simulink model "Laboratory_2_Stateflow"  (R2023b)
settings: Solver=FixedStepAuto  StartTime=0.0  StopTime=1200.0  FixedStep=0.1  RelTol=1e-3
libraries: SignalEditorBlockLib x1
settings Model: PacingRate=10  Creator=cosmi  LastModifiedBy=cosmi

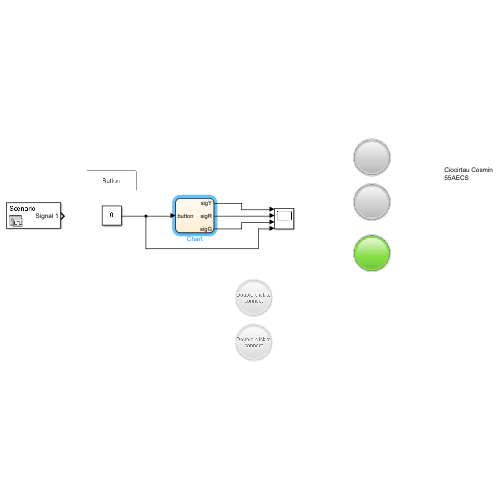
[thumbnail: Simulink's stored preview of the top-level diagram]
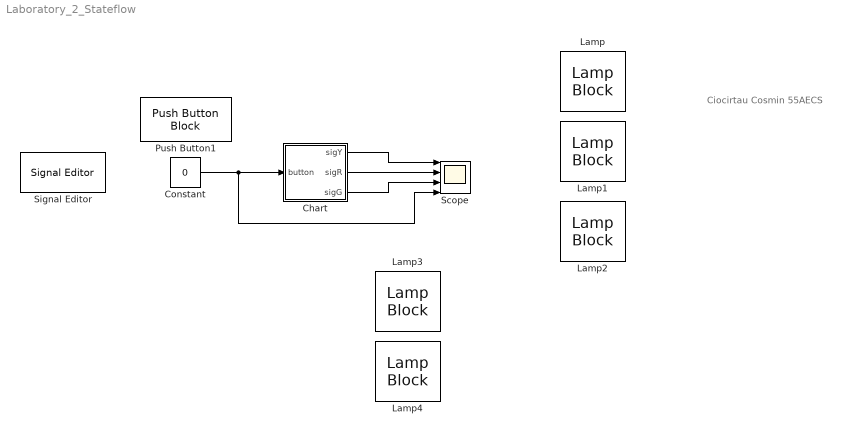
== system Laboratory_2_Stateflow ==
  note: Ciocirtau Cosmin
      | 55AECS
  Chart : Stateflow chart  TreatAsAtomicUnit=on
  Constant : Constant  Value=0
  Lamp{,1..4} (5 alike) : LampBlock  LabelPosition=Hide
  Push Button1 : PushButtonBlock  OffValue=0.000000
  Scope : Scope  NumInputPorts=4
  Signal Editor : SignalEditorBlockLib/Signal Editor  FileName=signal1.mat  ActiveScenario=Scenario  ActiveSignal=Signal 1  IsBus=off  OutputBusObjectStr=Bus: BusObject  SampleTime=0  Interpolate=off  ZeroCross=off  OutputAfterFinalValue=Setting to zero  Unit=inherit  PreserveSignalName=on  ApplySigPropsToAllScenarios=on  ApplySigPropsToAllSignals=off
  wires:
  Chart/3(sigG) -> Scope/3
  Chart/2(sigR) -> Scope/2
  Chart/1(sigY) -> Scope/1
  Constant/1 -> Scope/4, Chart/1(button)

== stateflow chart Laboratory_2_Stateflow/Chart ==
  state RED
  note: Ciocirtau Cosmin
      | 55AECS
  state Yellow
  state GREEN
  state WAIT
  (default) -> RED : {sigR = true;
      | sigY = false;
      | sigG = false}
  Yellow -> RED : [after(5,sec)]
      | {sigG = true;
      | sigR = false;
      | sigY = false;}
  RED -> GREEN : [after(30,sec)]/
      | {sigG = true;
      | sigR = false;
      | sigY = false;
      | count = 0;}
  GREEN -> GREEN [order 3] : {count = count + 1;}
  GREEN -> Yellow [order 1] : [button == true && count >= 600]/
      | {sigG = false;
      | sigR = false;
      | sigY = true;}
  WAIT -> Yellow [order 1] : [count >= 600]/{count = 0;
      | sigG = false;
      | sigR = false;
      | sigY = true;}
  GREEN -> WAIT [order 2] : [button == true]
  WAIT -> WAIT [order 2] : {count = count + 1;}
  data: count local; sigY output; sigR output; sigG output; button input
